simulink library "common_lib"  (R2023a)
settings: Solver=ode45  StartTime=0.0  StopTime=10.0  RelTol=1e-3
undefined symbols (not defined in the file): ACCEL_PRE_MULT, APDT_SrvcMgr_IRVHVDCSubFcnReq, C_C1GearNumbers, C_C1GearRatios, C_Calibration, C_DitherWaveform, C_GearOffset, C_GearRatioIn, C_GearRatioInverseOut, C_GearRatioOut, CLUTCH_INNER_LOOP_UPDATE_RATE, CONSTANT, DEGRADED_MODE_SIZE, Dem_EventStatusType, DiscIntNeverNeededParam, F_FAULT_ENUM, F_NOFAULT, F_OUTOFRANGE, F_RATELIMIT, FALSE, FMI14_SPECIAL_INSTRUCTIONS, FMI20_DATA_DRIFTED_HIGH, FMI21_DATA_DRIFTED_LOW, FMI29_RESERVED_FOR_SAE_ASSIGNMENT, FMI30_RESERVED_FOR_SAE_ASSIGNMENT, FMI31_CONDITION_EXISTS, FMI32_NO_FAULT, IC, k_accel, k_mean, MAX_UINT32, MEAN_PRE_MULT, NTriggers, QLTY_SIGNAL_FAILED, QLTY_SIGNAL_FULLY_FUNCTION, QLTY_SIGNAL_SUBSTITUTED_BY_1ST_CHOICE, QLTY_SIGNAL_SUBSTITUTED_BY_2ND_CHOICE, QLTY_SIGNAL_SUBSTITUTED_BY_3RD_CHOICE, QLTY_SIGNAL_SUBSTITUTED_BY_4TH_CHOICE, SAMPLE_TIME_100us, SAMPLETIME_10ms_Int, SATURATION_U16, simin, T_TestPoint, TF_FALSE, TF_TRUE, TimeStep, TRUE, WORKSPACE_UPDATE_RATE, ZERO, Zero
libraries: $bdroot x123, simulink x28, simulink_extras x4, MBD_EPS_Local_Blockset x4
(part 10 of 10)

== system common_lib/Signal Generators/Signal Generator Components/TestSignalPeriod ==
  TestSignalFrequency : Inport
  ClampAboveZero : $bdroot/Misc/ClampAboveZero  Tol=single(0.0001)
      settings: AttributesFormatString=tol=%<Tol>
  ClampAroundZero1 : $bdroot/Misc/ClampAroundZero  Tol=single(0.01)
      settings: AttributesFormatString=tol=%<Tol>
  Constant1 : Constant  Value=TimeStep  SampleTime=-1
  Constant35 : Constant  Value=single(2.0)  SampleTime=-1
  Constant39 : Constant  Value=single(1.0)  SampleTime=-1
  Data Type Conversion1 : DataTypeConversion  OutDataTypeStr=single  SaturateOnIntegerOverflow=off  RndMeth=Floor
  MinMax1 : MinMax  Function=max  Inputs=2  InputSameDT=on  ZeroCross=off
  Product15 : Product  Inputs=*/  OutDataTypeStr=Inherit: Same as first input
  Product19 : Product  Inputs=**  InputSameDT=on  OutDataTypeStr=Inherit: Same as first input
  TestSignalPeriod : Outport  VectorParamsAs1DForOutWhenUnconnected=off
  wires:
  Product15/1 -> MinMax1/1
  Constant39/1 -> Product15/1
  ClampAroundZero1/1 -> Product15/2
  TestSignalFrequency/1 -> ClampAroundZero1/1
  Constant1/1 -> Data Type Conversion1/1
  Constant35/1 -> Product19/2
  Product19/1 -> MinMax1/2
  MinMax1/1 -> TestSignalPeriod/1  "TestSignalPeriod"
  ClampAboveZero/1 -> Product19/1
  Data Type Conversion1/1 -> ClampAboveZero/1

== system common_lib/Signal Generators/Signal Generator Components/TestSignalPeriodTimer ==
  TestSignalReset : Inport
  TestSignalPeriod : Inport  Port=2
  ClampAboveZero : $bdroot/Misc/ClampAboveZero  Tol=single(0.0001)
      settings: AttributesFormatString=tol=%<Tol>
  Constant1 : Constant  Value=TimeStep  SampleTime=-1
  Constant40 : Constant  Value=false  SampleTime=-1
  Constant41 : Constant  Value=single(0.0)
  Data Type Conversion7 : DataTypeConversion  OutDataTypeStr=single  SaturateOnIntegerOverflow=off  RndMeth=Floor
  Logical Operator1 : Logic  Operator=OR  Inputs=3  AllPortsSameDT=off
  Relational Operator4 : RelationalOperator  ZeroCross=off  InputSameDT=off
  Sum5 : Sum  Inputs=2
  Switch5 : Switch  Threshold=0.5  ZeroCross=off  SaturateOnIntegerOverflow=off  InputSameDT=off
  Unit Delay4 : UnitDelay  InitialCondition=true  SampleTime=-1  HasFrameUpgradeWarning=on
      settings: AttributesFormatString=ic=%<X0>
  Unit Delay5 : UnitDelay  InitialCondition=single(0.0)  SampleTime=-1  HasFrameUpgradeWarning=on
      settings: AttributesFormatString=ic=%<X0>
  TestSignalTime : Outport  VectorParamsAs1DForOutWhenUnconnected=off
  wires:
  TestSignalReset/1 -> Logical Operator1/2
  Logical Operator1/1 -> Switch5/2
  Switch5/1 -> Unit Delay5/1, TestSignalTime/1  "TestSignalTime"
  Sum5/1 -> Switch5/3
  Constant41/1 -> Switch5/1
  Unit Delay4/1 -> Logical Operator1/1
  Constant40/1 -> Unit Delay4/1
  TestSignalPeriod/1 -> Relational Operator4/2
  Relational Operator4/1 -> Logical Operator1/3
  Unit Delay5/1 -> Relational Operator4/1, Sum5/1
  Constant1/1 -> Data Type Conversion7/1
  Data Type Conversion7/1 -> ClampAboveZero/1
  ClampAboveZero/1 -> Sum5/2

== system common_lib/Signal Generators/Signal Generator Components/TestSignalRamp ==
  TestSignalRampStart : Inport
  TestSignalRampEnd : Inport  Port=2
  TestSignalRampTime : Inport  Port=3
  TestSignalReset : Inport  Port=4
  Abs : Abs  ZeroCross=off  SaturateOnIntegerOverflow=off
  Constant35 : Constant  Value=single(0.01)  SampleTime=-1
  Logical Operator : Logic  AllPortsSameDT=off
  Logical Operator1 : Logic  Operator=NOT  AllPortsSameDT=off
  Logical Operator2 : Logic  Operator=NOT  AllPortsSameDT=off
  Logical Operator3 : Logic  Operator=OR  AllPortsSameDT=off
  Relational Operator : RelationalOperator  ZeroCross=off  InputSameDT=off
  Sum : Sum  Inputs=+-
  TestSignalRampEnabled : Subsystem
  Unit Delay : UnitDelay  InitialCondition=CLUTCH_INNER_LOOP_UPDATE_RATE  SampleTime=-1  HasFrameUpgradeWarning=on
      settings: AttributesFormatString=ic=%<X0>
  TestSignal : Outport  VectorParamsAs1DForOutWhenUnconnected=off
  wires:
  Logical Operator3/1 -> Logical Operator/2
  Logical Operator2/1 -> Logical Operator3/2
  Unit Delay/1 -> Logical Operator2/1
  Logical Operator1/1 -> Logical Operator3/1
  Logical Operator/1 -> TestSignalRampEnabled/Enable
  Relational Operator/1 -> Logical Operator/1
  Constant35/1 -> Relational Operator/2
  Abs/1 -> Relational Operator/1
  Sum/1 -> Abs/1
  TestSignalRampTime/1 -> TestSignalRampEnabled/3(TestSignalFreqRampTime)
  TestSignalRampEnabled/1(TestSignalFrequency) -> TestSignal/1
  TestSignalRampEnd/1 -> Sum/2, TestSignalRampEnabled/2(TestSignalFreqRampEnd)
  TestSignalRampStart/1 -> Sum/1, TestSignalRampEnabled/1(TestSignalFrequencyIn)
  TestSignalReset/1 -> Unit Delay/1, Logical Operator1/1, TestSignalRampEnabled/4(TestSignalReset)

== system common_lib/Signal Generators/Signal Generator Components/TestSignalSineWave ==
  TestSignalPk2PkAmplitude : Inport
  TestSignalOffset : Inport  Port=2
  TestSignalTime : Inport  Port=3
  TestSignalPeriod : Inport  Port=4
  TestSignalReset : Inport  Port=5
  Constant1 : Constant  Value=single(0.0)
  Data Type Conversion4 : DataTypeConversion  OutDataTypeStr=uint32  SaturateOnIntegerOverflow=off
  Look-Up Table : Lookup  InputValues=single([0 0.25 0.5 0.75 1])  Table=single([0 pi/2 0 -pi/2 0])  LookUpMeth=Interpolation-Use End Values  SaturateOnIntegerOverflow=off
      settings: AttributesFormatString=X=%<InputValues>\nY= %<OutputValues>
  Product1 : Product  Inputs=*/  OutDataTypeStr=Inherit: Same as first input
  Product16 : Product  Inputs=*/  OutDataTypeStr=Inherit: Same as first input
  Product18 : Product  Inputs=**  OutDataTypeStr=Inherit: Same as first input
  Sine1 : $bdroot/Misc/Sine
  Sum3 : Sum  Inputs=+-
  Sum4 : Sum
  Switch1 : Switch  Threshold=0.5  ZeroCross=off  SaturateOnIntegerOverflow=off  InputSameDT=off
  TestSignal : Outport  VectorParamsAs1DForOutWhenUnconnected=off
  wires:
  Sine1/1 -> Product18/1
  Look-Up Table/1 -> Sine1/1
  Product1/1 -> Look-Up Table/1  "TestSignalPeriodFrac"
  [TestSignalPeriod] -> Product1/2
  Switch1/1 -> Sum4/1
  Constant1/1 -> Switch1/1
  TestSignalReset/1 -> Switch1/2
  TestSignalPk2PkAmplitude/1 -> Product18/2
  TestSignalOffset/1 -> Sum4/2
  Sum4/1 -> TestSignal/1  "TestSignal"
  Product16/1 -> Sum3/1, Data Type Conversion4/1
  Data Type Conversion4/1 -> Sum3/2
  Sum3/1 -> Product1/1
  Product18/1 -> Switch1/3
  TestSignalTime/1 -> Product16/1, [TestSignalTime]
  TestSignalPeriod/1 -> Product16/2, [TestSignalPeriod]

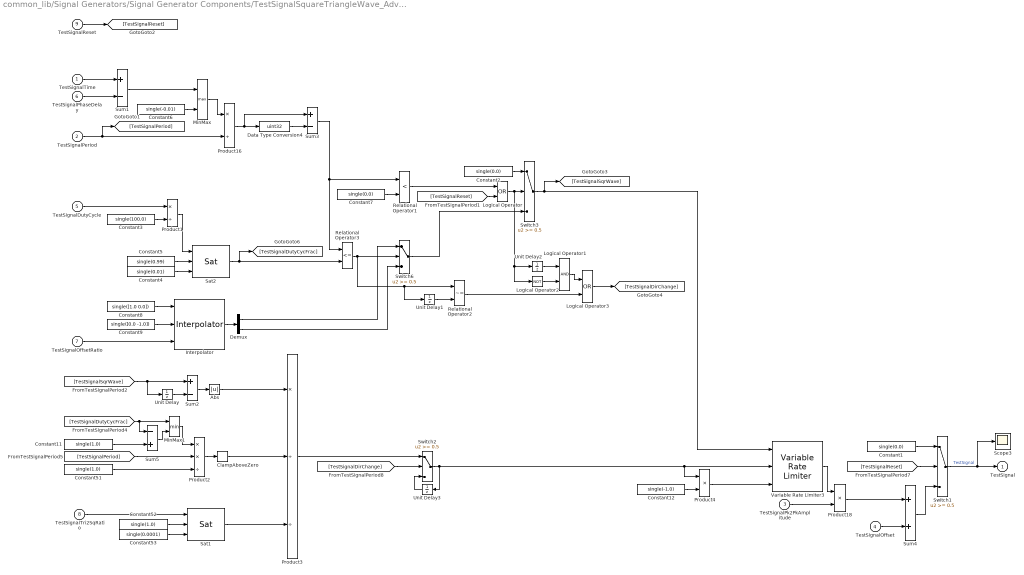
== system common_lib/Signal Generators/Signal Generator Components/TestSignalSquareTriangleWave_Advanced ==
  TestSignalTime : Inport
  TestSignalPeriod : Inport  Port=2
  TestSignalPk2PkAmplitude : Inport  Port=3
  TestSignalOffset : Inport  Port=4
  TestSignalDutyCycle : Inport  Port=5
  TestSignalPhaseDelay : Inport  Port=6
  TestSignalOffsetRatio : Inport  Port=7
  TestSignalTri2SqRatio : Inport  Port=8
  TestSignalReset : Inport  Port=9
  Abs : Abs  ZeroCross=off  SaturateOnIntegerOverflow=off
  ClampAboveZero : $bdroot/Misc/ClampAboveZero  Tol=single(0.001)
      settings: AttributesFormatString=tol=%<Tol>
  Constant1 : Constant  Value=single(0.0)
  Constant11 : Constant  Value=single(1.0)
  Constant12 : Constant  Value=single(-1.0)
  Constant2 : Constant  Value=single(0.0)
  Constant3 : Constant  Value=single(100.0)
  Constant4 : Constant  Value=single(0.01)
  Constant5 : Constant  Value=single(0.99)
  Constant51 : Constant  Value=single(1.0)
  Constant52 : Constant  Value=single(1.0)
  Constant53 : Constant  Value=single(0.0001)
  Constant6 : Constant  Value=single(-0.01)
  Constant7 : Constant  Value=single(0.0)
  Constant8 : Constant  Value=single([1.0 0.0])
  Constant9 : Constant  Value=single([0.0 -1.0])
  Data Type Conversion4 : DataTypeConversion  OutDataTypeStr=uint32  SaturateOnIntegerOverflow=off
  Demux : Demux  Outputs=2
  Interpolator : $bdroot/Tbl/Interpolator  DType=Single
  Logical Operator : Logic  Operator=OR  AllPortsSameDT=off
  Logical Operator1 : Logic  AllPortsSameDT=off
  Logical Operator2 : Logic  Operator=NOT  AllPortsSameDT=off
  Logical Operator3 : Logic  Operator=OR  AllPortsSameDT=off
  MinMax : MinMax  Function=max  Inputs=2  InputSameDT=on  ZeroCross=off
  MinMax1 : MinMax  Inputs=2  InputSameDT=on  ZeroCross=off
  Product1 : Product  Inputs=*/  OutDataTypeStr=Inherit: Same as first input
  Product16 : Product  Inputs=*/  OutDataTypeStr=Inherit: Same as first input
  Product18 : Product  Inputs=**  OutDataTypeStr=Inherit: Same as first input
  Product2 : Product  Inputs=**/  OutDataTypeStr=Inherit: Same as first input
  Product3 : Product  Inputs=*//  OutDataTypeStr=Inherit: Same as first input
  Product4 : Product  Inputs=**  OutDataTypeStr=Inherit: Same as first input
  Relational Operator1 : RelationalOperator  Operator=<  ZeroCross=off  InputSameDT=off
  Relational Operator2 : RelationalOperator  Operator=~=  ZeroCross=off  InputSameDT=off
  Relational Operator3 : RelationalOperator  Operator=<=  ZeroCross=off  InputSameDT=off
  Sat1 : $bdroot/Slink/Sat
  Sat2 : $bdroot/Slink/Sat
  Scope3 : Scope
  Sum1 : Sum  Inputs=+-
  Sum2 : Sum  Inputs=+-
  Sum3 : Sum  Inputs=+-
  Sum4 : Sum
  Sum5 : Sum  Inputs=-+
  Switch{1..3,6} (4 alike) : Switch  Threshold=0.5  ZeroCross=off  SaturateOnIntegerOverflow=off  InputSameDT=off
  Unit Delay : UnitDelay  InitialCondition=single(0.0)  SampleTime=-1  HasFrameUpgradeWarning=on
      settings: AttributesFormatString=ic=%<X0>
  Unit Delay1 : UnitDelay  InitialCondition=false  SampleTime=-1  HasFrameUpgradeWarning=on
      settings: AttributesFormatString=ic=%<X0>
  Unit Delay2 : UnitDelay  InitialCondition=false  SampleTime=-1  HasFrameUpgradeWarning=on
      settings: AttributesFormatString=ic=%<X0>
  Unit Delay3 : UnitDelay  InitialCondition=single(0.0)  SampleTime=-1  HasFrameUpgradeWarning=on
      settings: AttributesFormatString=ic=%<X0>
  Variable Rate Limiter3 : $bdroot/Slink/Variable Rate Limiter  TimeStep=TimeStep  ic=single(0.0)
  TestSignal : Outport  VectorParamsAs1DForOutWhenUnconnected=off
  wires:
  MinMax1/1 -> Product2/1
  Product4/1 -> Variable Rate Limiter3/3
  Constant12/1 -> Product4/2
  Abs/1 -> Product3/1
  [TestSignalDirChange] -> Switch2/2
  Unit Delay3/1 -> Switch2/3
  Switch2/1 -> Unit Delay3/1, Product4/1, Variable Rate Limiter3/2
  [TestSignalReset] -> Switch1/2
  Product3/1 -> Switch2/1
  Sum5/1 -> MinMax1/2
  Constant11/1 -> Sum5/2
  ClampAboveZero/1 -> Product3/2
  Sum2/1 -> Abs/1
  Product2/1 -> ClampAboveZero/1
  [TestSignalPeriod] -> Product2/2
  [TestSignalDutyCycFrac] -> MinMax1/1, Sum5/1
  Unit Delay/1 -> Sum2/2
  Logical Operator3/1 -> [TestSignalDirChange]
  Relational Operator2/1 -> Logical Operator3/2
  Logical Operator1/1 -> Logical Operator3/1
  Logical Operator2/1 -> Logical Operator1/2
  Unit Delay2/1 -> Logical Operator1/1
  Unit Delay1/1 -> Relational Operator2/2
  [TestSignalSqrWave] -> Sum2/1, Unit Delay/1
  Logical Operator/1 -> Logical Operator2/1, Unit Delay2/1, Switch3/2
  [TestSignalReset] -> Logical Operator/2
  Demux/2 -> Switch6/3
  Demux/1 -> Switch6/1
  Interpolator/1 -> Demux/1
  Constant2/1 -> Switch3/1
  Constant8/1 -> Interpolator/1
  Switch3/1 -> [TestSignalSqrWave], Variable Rate Limiter3/1
  Constant9/1 -> Interpolator/2
  TestSignalOffsetRatio/1 -> Interpolator/3
  Relational Operator1/1 -> Logical Operator/1
  Constant7/1 -> Relational Operator1/2
  MinMax/1 -> Product16/1
  Constant6/1 -> MinMax/2
  TestSignalPhaseDelay/1 -> Sum1/2
  Sum1/1 -> MinMax/1
  Sat2/1 -> [TestSignalDutyCycFrac], Relational Operator3/2
  Constant5/1 -> Sat2/2
  Constant4/1 -> Sat2/3
  Product1/1 -> Sat2/1
  Constant3/1 -> Product1/2
  TestSignalDutyCycle/1 -> Product1/1
  Switch1/1 -> Scope3/1, TestSignal/1  "TestSignal"
  Constant1/1 -> Switch1/1
  Sat1/1 -> Product3/3
  Constant53/1 -> Sat1/3
  Constant52/1 -> Sat1/2
  TestSignalTri2SqRatio/1 -> Sat1/1
  Constant51/1 -> Product2/3
  Variable Rate Limiter3/1 -> Product18/1
  TestSignalPk2PkAmplitude/1 -> Product18/2
  TestSignalOffset/1 -> Sum4/2
  Product16/1 -> Sum3/1, Data Type Conversion4/1
  Data Type Conversion4/1 -> Sum3/2
  Sum3/1 -> Relational Operator1/1, Relational Operator3/1
  Relational Operator3/1 -> Unit Delay1/1, Relational Operator2/1, Switch6/2
  Switch6/1 -> Switch3/3
  Product18/1 -> Sum4/1
  TestSignalTime/1 -> Sum1/1
  TestSignalPeriod/1 -> Product16/2, [TestSignalPeriod]
  Sum4/1 -> Switch1/3
  TestSignalReset/1 -> [TestSignalReset]

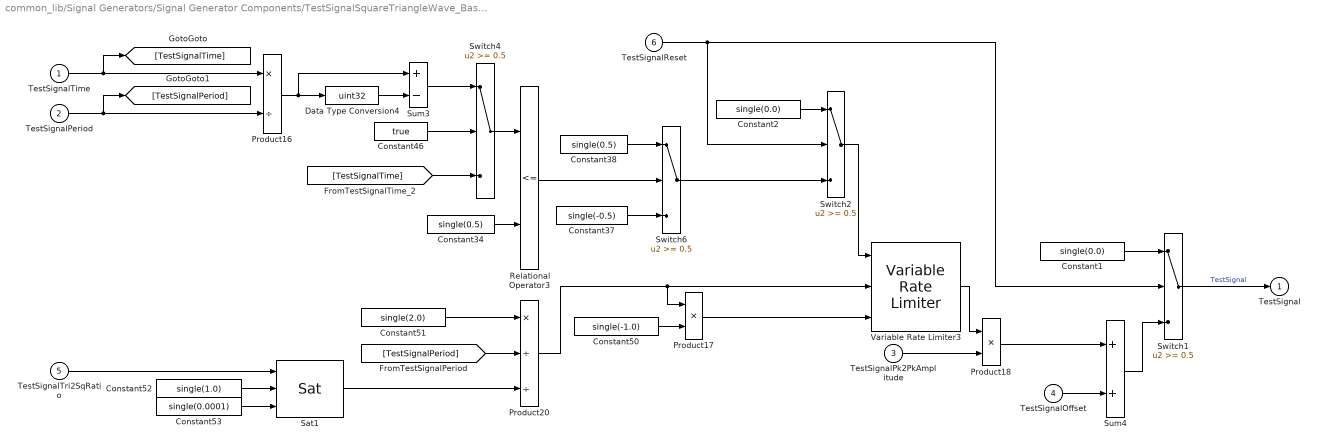
== system common_lib/Signal Generators/Signal Generator Components/TestSignalSquareTriangleWave_Basic ==
  TestSignalTime : Inport
  TestSignalPeriod : Inport  Port=2
  TestSignalPk2PkAmplitude : Inport  Port=3
  TestSignalOffset : Inport  Port=4
  TestSignalTri2SqRatio : Inport  Port=5
  TestSignalReset : Inport  Port=6
  Constant1 : Constant  Value=single(0.0)
  Constant2 : Constant  Value=single(0.0)
  Constant34 : Constant  Value=single(0.5)  SampleTime=-1
  Constant37 : Constant  Value=single(-0.5)  SampleTime=-1
  Constant38 : Constant  Value=single(0.5)  SampleTime=-1
  Constant46 : Constant  Value=true  SampleTime=-1
  Constant50 : Constant  Value=single(-1.0)
  Constant51 : Constant  Value=single(2.0)
  Constant52 : Constant  Value=single(1.0)
  Constant53 : Constant  Value=single(0.0001)
  Data Type Conversion4 : DataTypeConversion  OutDataTypeStr=uint32  SaturateOnIntegerOverflow=off
  Product16 : Product  Inputs=*/  OutDataTypeStr=Inherit: Same as first input
  Product17 : Product  Inputs=**  OutDataTypeStr=Inherit: Same as first input
  Product18 : Product  Inputs=**  OutDataTypeStr=Inherit: Same as first input
  Product20 : Product  Inputs=*//  OutDataTypeStr=Inherit: Same as first input
  Relational Operator3 : RelationalOperator  Operator=<=  ZeroCross=off  InputSameDT=off
  Sat1 : $bdroot/Slink/Sat
  Sum3 : Sum  Inputs=+-
  Sum4 : Sum
  Switch{1..2,4,6} (4 alike) : Switch  Threshold=0.5  ZeroCross=off  SaturateOnIntegerOverflow=off  InputSameDT=off
  Variable Rate Limiter3 : $bdroot/Slink/Variable Rate Limiter  TimeStep=TimeStep  ic=single(0.0)
  TestSignal : Outport  VectorParamsAs1DForOutWhenUnconnected=off
  wires:
  Switch2/1 -> Variable Rate Limiter3/1
  Constant2/1 -> Switch2/1
  TestSignalReset/1 -> Switch1/2, Switch2/2
  Sum4/1 -> Switch1/3
  TestSignalPeriod/1 -> [TestSignalPeriod], Product16/2
  TestSignalTime/1 -> [TestSignalTime], Product16/1
  Product18/1 -> Sum4/1
  Switch6/1 -> Switch2/3
  Constant38/1 -> Switch6/1
  Constant37/1 -> Switch6/3
  Relational Operator3/1 -> Switch6/2
  Switch4/1 -> Relational Operator3/1
  [TestSignalTime] -> Switch4/3
  Constant46/1 -> Switch4/2
  Sum3/1 -> Switch4/1
  Data Type Conversion4/1 -> Sum3/2
  Product16/1 -> Data Type Conversion4/1, Sum3/1
  Constant34/1 -> Relational Operator3/2
  TestSignalOffset/1 -> Sum4/2
  TestSignalPk2PkAmplitude/1 -> Product18/2
  Product20/1 -> Product17/1, Variable Rate Limiter3/2
  Product17/1 -> Variable Rate Limiter3/3
  Constant50/1 -> Product17/2
  Variable Rate Limiter3/1 -> Product18/1
  Constant51/1 -> Product20/1
  [TestSignalPeriod] -> Product20/2
  TestSignalTri2SqRatio/1 -> Sat1/1
  Constant52/1 -> Sat1/2
  Constant53/1 -> Sat1/3
  Sat1/1 -> Product20/3
  Constant1/1 -> Switch1/1
  Switch1/1 -> TestSignal/1  "TestSignal"

== system common_lib/Signal Generators/Signal Generator Components/TestSignalTimer ==
  TestSignalReset : Inport
  Constant1 : Constant  Value=TimeStep  SampleTime=-1
  Constant40 : Constant  Value=false  SampleTime=-1
  Constant41 : Constant  Value=single(0.0)
  Constant43 : Constant  Value=single(1000000)
  Data Type Conversion7 : DataTypeConversion  OutDataTypeStr=single  SaturateOnIntegerOverflow=off  RndMeth=Floor
  Logical Operator1 : Logic  Operator=OR  Inputs=3  AllPortsSameDT=off
  Relational Operator4 : RelationalOperator  ZeroCross=off  InputSameDT=off
  Sum5 : Sum  Inputs=2
  Switch5 : Switch  Threshold=0.5  ZeroCross=off  SaturateOnIntegerOverflow=off  InputSameDT=off
  Unit Delay4 : UnitDelay  InitialCondition=true  SampleTime=-1  HasFrameUpgradeWarning=on
      settings: AttributesFormatString=ic=%<X0>
  Unit Delay5 : UnitDelay  InitialCondition=single(0.0)  SampleTime=-1  HasFrameUpgradeWarning=on
      settings: AttributesFormatString=ic=%<X0>
  TestSignalTime : Outport  VectorParamsAs1DForOutWhenUnconnected=off
  wires:
  Constant1/1 -> Data Type Conversion7/1
  TestSignalReset/1 -> Logical Operator1/2
  Logical Operator1/1 -> Switch5/2
  Switch5/1 -> Unit Delay5/1, TestSignalTime/1  "TestSignalTime"
  Sum5/1 -> Switch5/3
  Constant41/1 -> Switch5/1
  Unit Delay4/1 -> Logical Operator1/1
  Constant40/1 -> Unit Delay4/1
  Constant43/1 -> Relational Operator4/2
  Relational Operator4/1 -> Logical Operator1/3
  Unit Delay5/1 -> Relational Operator4/1, Sum5/1
  Data Type Conversion7/1 -> Sum5/2

== system common_lib/Tbl/XY Interpolator1/XYInterp ==
  y_value_1 : Inport
  y_value_0 : Inport  Port=2
  x_value_1 : Inport  Port=3
  x_value_0 : Inport  Port=4
  x_value : Inport  Port=5
  ClampAroundZero : $bdroot/Misc/ClampAroundZero  Tol=Tol
  Constant1 : Constant  Value=Zero
  Constant2 : Constant  Value=One
  Product1 : Product  Inputs=*/  InputSameDT=on  OutDataTypeStr=Inherit: Same as first input
  Product2 : Product  Inputs=**  InputSameDT=on  OutDataTypeStr=Inherit: Same as first input
  Sat : $bdroot/Slink/Sat
  Sum : Sum  Inputs=+-  InputSameDT=on  OutDataTypeStr=Inherit: Same as first input
  Sum1 : Sum  Inputs=|++  InputSameDT=on  OutDataTypeStr=Inherit: Same as first input
  Sum2 : Sum  Inputs=-+  InputSameDT=on  OutDataTypeStr=Inherit: Same as first input
  Sum3 : Sum  Inputs=+-  InputSameDT=on  OutDataTypeStr=Inherit: Same as first input
  output : Outport  VectorParamsAs1DForOutWhenUnconnected=off
  wires:
  y_value_0/1 -> Sum1/2, Sum/2
  y_value_1/1 -> Sum/1
  Sum1/1 -> output/1
  Product2/1 -> Sum1/1
  Sum/1 -> Product2/1
  x_value/1 -> Sum3/1
  x_value_0/1 -> Sum3/2, Sum2/1
  Sum3/1 -> Product1/1
  x_value_1/1 -> Sum2/2
  Sum2/1 -> ClampAroundZero/1
  ClampAroundZero/1 -> Product1/2
  Product1/1 -> Sat/1
  Sat/1 -> Product2/2
  Constant2/1 -> Sat/2
  Constant1/1 -> Sat/3

== system common_lib/Diagnostics/Calibration Enabled MinMax OOR/Enabled OOR/OOR MinMax Capture ==
  Input : Inport
  Hold : Inport  Port=2
  Enable : EnablePort  ZeroCross=off
  CL MinMax Capture : $bdroot/Diag/CL MinMax Capture  CaptureType=Max  InDataType=single
  CL MinMax Capture1 : $bdroot/Diag/CL MinMax Capture  CaptureType=Min  InDataType=single
  DRDataStoreRead : DataStoreRead  DataStoreName=InitializeStates  IndexOptions=Index vector (dialog)  Indices=1  OutputSizes=1
  Max : Outport  VectorParamsAs1DForOutWhenUnconnected=off
  Min : Outport  Port=2  VectorParamsAs1DForOutWhenUnconnected=off
  wires:
  Input/1 -> CL MinMax Capture1/1, CL MinMax Capture/1
  Hold/1 -> CL MinMax Capture1/2, CL MinMax Capture/2
  DRDataStoreRead/1 -> CL MinMax Capture/3, CL MinMax Capture1/3
  CL MinMax Capture/1 -> Max/1
  CL MinMax Capture1/1 -> Min/1

== system common_lib/Diagnostics/Calibration Enabled MinMax RLim/Enabled RLim/RLim MinMax Capture ==
  Input : Inport
  Hold : Inport  Port=2
  Enable : EnablePort  ZeroCross=off
  CL MinMax Capture : $bdroot/Diag/CL MinMax Capture  CaptureType=Max  InDataType=single
  CL MinMax Capture1 : $bdroot/Diag/CL MinMax Capture  CaptureType=Min  InDataType=single
  DRDataStoreRead : DataStoreRead  DataStoreName=InitializeStates  IndexOptions=Index vector (dialog)  Indices=1  OutputSizes=1
  Sum1 : Sum  Inputs=|+-  InputSameDT=on  OutDataTypeStr=Inherit: Same as first input
  Unit Delay2 : UnitDelay  InitialCondition=Zero  SampleTime=-1  HasFrameUpgradeWarning=on
      settings: AttributesFormatString=ic=%<X0>
  Max : Outport  VectorParamsAs1DForOutWhenUnconnected=off
  Min : Outport  Port=2  VectorParamsAs1DForOutWhenUnconnected=off
  wires:
  Input/1 -> Sum1/1, Unit Delay2/1
  Hold/1 -> CL MinMax Capture1/2, CL MinMax Capture/2
  CL MinMax Capture/1 -> Max/1
  CL MinMax Capture1/1 -> Min/1
  Unit Delay2/1 -> Sum1/2
  Sum1/1 -> CL MinMax Capture1/1, CL MinMax Capture/1
  DRDataStoreRead/1 -> CL MinMax Capture/3, CL MinMax Capture1/3

== system common_lib/Diagnostics/Calibration Enabled MinMax RLim/Enabled RLim/RateLimit ==
  in : Inport
  rlim : Inport  Port=2
  ext_fault? : Inport  Port=3
  Constant2 : Constant  Value=TimeStep
  DRDataStoreRead : DataStoreRead  DataStoreName=InitializeStates  IndexOptions=Index vector (dialog)  Indices=1  OutputSizes=1
  Data Type Conversion : DataTypeConversion  OutDataTypeStr=single  SaturateOnIntegerOverflow=off  RndMeth=Floor
  Logical Operator : Logic  Operator=NOT
  OOR Fault Detection : $bdroot/Diag/OOR Fault Detection  InitialValue=IC
  Product1 : Product  InputSameDT=on  OutDataTypeStr=Inherit: Same as first input
  Sum1 : Sum  Inputs=-+|  InputSameDT=on  OutDataTypeStr=Inherit: Same as first input
  Sum2 : Sum  Inputs=|++  InputSameDT=on  OutDataTypeStr=Inherit: Same as first input
  Sum3 : Sum  Inputs=++|  InputSameDT=on  OutDataTypeStr=Inherit: Same as first input
  Unit Delay : UnitDelay  InitialCondition=Zero  SampleTime=-1  HasFrameUpgradeWarning=on
      settings: AttributesFormatString=ic=%<X0>
  Unit Delay1 : UnitDelay  InitialCondition=false  SampleTime=-1  HasFrameUpgradeWarning=on
      settings: AttributesFormatString=ic=%<X0>
  Unit Delay2 : UnitDelay  InitialCondition=Zero  SampleTime=-1  HasFrameUpgradeWarning=on
      settings: AttributesFormatString=ic=%<X0>
  inc switch : Switch  Threshold=0.5  ZeroCross=off  SaturateOnIntegerOverflow=off
  inc switch1 : Switch  Threshold=0.5  ZeroCross=off  SaturateOnIntegerOverflow=off
  out : Outport  VectorParamsAs1DForOutWhenUnconnected=off
  fault? : Outport  Port=2  VectorParamsAs1DForOutWhenUnconnected=off
  wires:
  Constant2/1 -> Data Type Conversion/1
  Data Type Conversion/1 -> Product1/1
  inc switch1/1 -> Sum2/1, Sum1/2
  Unit Delay/1 -> inc switch1/1
  Unit Delay1/1 -> inc switch/2
  Unit Delay2/1 -> Sum3/1
  Sum3/1 -> inc switch/1
  Product1/1 -> Sum3/2, inc switch/3
  rlim/1 -> Product1/2
  inc switch/1 -> Unit Delay2/1, Sum1/1, Sum2/2
  Sum2/1 -> OOR Fault Detection/2
  Sum1/1 -> OOR Fault Detection/3
  OOR Fault Detection/2 -> Unit Delay1/1, fault?/1
  OOR Fault Detection/1 -> Unit Delay/1, out/1
  ext_fault?/1 -> OOR Fault Detection/4
  in/1 -> inc switch1/3, OOR Fault Detection/1
  DRDataStoreRead/1 -> Logical Operator/1
  Logical Operator/1 -> inc switch1/2

== system common_lib/OS/Scheduler with Init/Init Relay/Function Call ==
  InitActive : EnablePort  StatesWhenEnabling=reset  ZeroCross=off
  Function-Call Generator : simulink/Ports & Subsystems/Function-Call Generator  sample_time=-1  numberOfIterations=1  DisallowWideOutput=off
  Init : Outport  VectorParamsAs1DForOutWhenUnconnected=off
  wires:
  Function-Call Generator/1 -> Init/1

== system common_lib/Signal Generators/Signal Generator Components/TestSignalRamp/TestSignalRampEnabled ==
  TestSignalFrequencyIn : Inport
  TestSignalFreqRampEnd : Inport  Port=2
  TestSignalFreqRampTime : Inport  Port=3
  TestSignalReset : Inport  Port=4
  Enable : EnablePort  StatesWhenEnabling=reset  ZeroCross=off
  Ramp : $bdroot/Ctrl/Ramp  TimeStep=TimeStep
  TestSignalFrequency : Outport  VectorParamsAs1DForOutWhenUnconnected=off
  wires:
  Ramp/1 -> TestSignalFrequency/1
  TestSignalReset/1 -> Ramp/4
  TestSignalFreqRampTime/1 -> Ramp/3
  TestSignalFreqRampEnd/1 -> Ramp/2
  TestSignalFrequencyIn/1 -> Ramp/1

== stateflow chart common_lib/Bit/uint8 Bit Pack ==
  settings: stateMachineType=MEALY_MACHINE
  (default) -> (junction 10) : {Byte=0;}
  (junction 10) -> (junction 13) [order 1] : [Bit_0]{Byte=Byte | 1;}
  (junction 10) -> (junction 13) [order 2]
  (junction 13) -> (junction 20) [order 1] : [Bit_1]{Byte=Byte | 2;}
  (junction 13) -> (junction 20) [order 2]
  (junction 20) -> (junction 26) [order 1] : [Bit_2]{Byte=Byte | 4;}
  (junction 20) -> (junction 26) [order 2]
  (junction 26) -> (junction 31) [order 1] : [Bit_3]{Byte=Byte | 8;}
  (junction 26) -> (junction 31) [order 2]
  (junction 31) -> (junction 36) [order 1] : [Bit_4]{Byte=Byte | 16;}
  (junction 31) -> (junction 36) [order 2]
  (junction 36) -> (junction 41) [order 1] : [Bit_5]{Byte=Byte | 32;}
  (junction 36) -> (junction 41) [order 2]
  (junction 41) -> (junction 46) [order 1] : [Bit_6]{Byte=Byte | 64;}
  (junction 41) -> (junction 46) [order 2]
  (junction 46) -> (junction 51) [order 1] : [Bit_7]{Byte=Byte | 128;}
  (junction 46) -> (junction 51) [order 2]
  data: Bit_0 input boolean size=1; Bit_1 input boolean size=1; Bit_2 input boolean size=1; Bit_3 input boolean size=1; Bit_4 input boolean size=1; Bit_5 input boolean size=1; Bit_6 input boolean size=1; Bit_7 input boolean size=1; Byte output uint8 size=1

== stateflow chart common_lib/Bit/uint8 Bit Unpack ==
  settings: stateMachineType=MEALY_MACHINE
  (default) -> (junction 17) : {Bit_0 = Byte & 1;
      |  Bit_1 = Byte & 2;
      |  Bit_2 = Byte & 4;
      |  Bit_3 = Byte & 8;
      |  Bit_4 = Byte & 16;
      |  Bit_5 = Byte & 32;
      |  Bit_6 = Byte & 64;
      |  Bit_7 = Byte & 128;}
  data: Byte input uint8 size=1; Bit_0 output boolean size=1; Bit_1 output boolean size=1; Bit_2 output boolean size=1; Bit_3 output boolean size=1; Bit_4 output boolean size=1; Bit_5 output boolean size=1; Bit_6 output boolean size=1; Bit_7 output boolean size=1

== stateflow chart common_lib/Bit/uint16 Bit Pack ==
  settings: stateMachineType=MEALY_MACHINE
  (default) -> (junction 10) : {Byte=0;}
  (junction 10) -> (junction 13) [order 1] : [Bit_0]{Byte=Byte | 1;}
  (junction 10) -> (junction 13) [order 2]
  (junction 13) -> (junction 20) [order 1] : [Bit_1]{Byte=Byte | 2;}
  (junction 13) -> (junction 20) [order 2]
  (junction 20) -> (junction 26) [order 1] : [Bit_2]{Byte=Byte | 4;}
  (junction 20) -> (junction 26) [order 2]
  (junction 26) -> (junction 31) [order 1] : [Bit_3]{Byte=Byte | 8;}
  (junction 26) -> (junction 31) [order 2]
  (junction 31) -> (junction 36) [order 1] : [Bit_4]{Byte=Byte | 16;}
  (junction 31) -> (junction 36) [order 2]
  (junction 36) -> (junction 41) [order 1] : [Bit_5]{Byte=Byte | 32;}
  (junction 36) -> (junction 41) [order 2]
  (junction 41) -> (junction 46) [order 1] : [Bit_6]{Byte=Byte | 64;}
  (junction 41) -> (junction 46) [order 2]
  (junction 46) -> (junction 65) [order 1] : [Bit_7]{Byte=Byte | 128;}
  (junction 46) -> (junction 65) [order 2]
  (junction 65) -> (junction 66) [order 1] : [Bit_8]{Byte=Byte | 256;}
  (junction 65) -> (junction 66) [order 2]
  (junction 66) -> (junction 69) [order 1] : [Bit_9]{Byte=Byte | 512;}
  (junction 66) -> (junction 69) [order 2]
  (junction 69) -> (junction 72) [order 1] : [Bit_10]{Byte=Byte | 1024;}
  (junction 69) -> (junction 72) [order 2]
  (junction 72) -> (junction 73) [order 1] : [Bit_11]{Byte=Byte | 2048;}
  (junction 72) -> (junction 73) [order 2]
  (junction 73) -> (junction 68) [order 1] : [Bit_12]{Byte=Byte | 4096;}
  (junction 73) -> (junction 68) [order 2]
  (junction 68) -> (junction 71) [order 1] : [Bit_13]{Byte=Byte | 8192;}
  (junction 68) -> (junction 71) [order 2]
  (junction 71) -> (junction 70) [order 1] : [Bit_14]{Byte=Byte | 16384;}
  (junction 71) -> (junction 70) [order 2]
  (junction 70) -> (junction 67) [order 1] : [Bit_15]{Byte=Byte | 32768;}
  (junction 70) -> (junction 67) [order 2]
  data: Bit_0 input boolean size=1; Bit_1 input boolean size=1; Bit_2 input boolean size=1; Bit_3 input boolean size=1; Bit_4 input boolean size=1; Bit_5 input boolean size=1; Bit_6 input boolean size=1; Bit_7 input boolean size=1; Byte output uint16 size=1; Bit_8 input boolean size=1; Bit_9 input boolean size=1; Bit_10 input boolean size=1; Bit_11 input boolean size=1; Bit_12 input boolean size=1; Bit_13 input boolean size=1; Bit_14 input boolean size=1; Bit_15 input boolean size=1

== stateflow chart common_lib/Bit/uint16 Bit Unpack ==
  settings: stateMachineType=MEALY_MACHINE
  (default) -> (junction 17) : {Bit_0 = Byte & 1;
      |  Bit_1 = Byte & 2;
      |  Bit_2 = Byte & 4;
      |  Bit_3 = Byte & 8;
      |  Bit_4 = Byte & 16;
      |  Bit_5 = Byte & 32;
      |  Bit_6 = Byte & 64;
      |  Bit_7 = Byte & 128;
      |  Bit_8 = Byte & 256;
      |  Bit_9 = Byte & 512;
      |  Bit_10 = Byte & 1024;
      |  Bit_11 = Byte & 2048;
      |  Bit_12 = Byte & 4096;
      |  Bit_13 = Byte & 8192;
      |  Bit_14 = Byte & 16384;
      |  Bit_15 = Byte & 32768;}
  data: Byte input uint16 size=1; Bit_0 output boolean size=1; Bit_1 output boolean size=1; Bit_2 output boolean size=1; Bit_3 output boolean size=1; Bit_4 output boolean size=1; Bit_5 output boolean size=1; Bit_6 output boolean size=1; Bit_7 output boolean size=1; Bit_8 output boolean size=1; Bit_9 output boolean size=1; Bit_10 output boolean size=1; Bit_11 output boolean size=1; Bit_12 output boolean size=1; Bit_13 output boolean size=1; Bit_14 output boolean size=1; Bit_15 output boolean size=1

== stateflow chart common_lib/Diagnostics/DiagFaultCounter/DiagFaulCounter ==
  state FaultDebounceDisabled
    en: diagFaultStatus = Dem_EventStatusType.DEM_EVENT_STATUS_INIT;
    diagFaultCnt = int16(0);
    FaultDebounceDisabled -> (junction 32) [order 1]
    (junction 32) -> (junction 29) [order 1] : [~diagStartUpComp || diagReset || ~diagEnable]
        | {diagFaultStatus = Dem_EventStatusType.DEM_EVENT_STATUS_INIT;}
    (junction 32) -> (junction 23) [order 2]
    (junction 29) -> (junction 27)
    (junction 23) -> (junction 24) [order 1] : [~diagFaultActive]
        | {diagFaultStatus = Dem_EventStatusType.DEM_EVENT_STATUS_PREPASSED;}
    (junction 23) -> (junction 26) [order 2]
    (junction 24) -> (junction 282)
    (junction 26) -> (junction 281) [order 1] : [diagFaultActive]
        | {diagFaultStatus = Dem_EventStatusType.DEM_EVENT_STATUS_PREFAILED;}
    (junction 26) -> (junction 51) [order 2]
    (junction 281) -> (junction 283)
    (junction 283) -> (junction 51)
    (junction 282) -> (junction 283)
    (junction 27) -> (junction 282)
    (junction 51) -> (junction 288)
  state FaultDebounceEnabled
    en: diagFaultStatus = Dem_EventStatusType.DEM_EVENT_STATUS_INIT;
    diagFaultCnt = int16(0);
    state Init
      en: diagFaultCnt = int16(0);
      diagFaultStatus = Dem_EventStatusType.DEM_EVENT_STATUS_INIT;
      Init -> (junction 248) [order 1]
      (junction 248) -> (junction 249) [order 1] : [~diagStartUpComp || diagReset || ~diagEnable]
          | {diagFaultCnt = int16(0);}
      (junction 248) -> (junction 250) [order 2]
      (junction 249) -> (junction 257)
      (junction 250) -> (junction 253) [order 1] : [~diagFaultActive]
          | {diagFaultCnt = diagFaultCnt - diagDnCnt;}
      (junction 253) -> (junction 342) [order 1] : [diagFaultCnt<=diagPassCntThresh]
          | {diagFaultStatus = Dem_EventStatusType.DEM_EVENT_STATUS_PASSED;}
      (junction 250) -> (junction 252) [order 2]
      (junction 253) -> (junction 255) [order 2]
      (junction 342) -> (junction 344)
      (junction 252) -> (junction 251) [order 1] : [diagFaultActive]
          | {diagFaultCnt = diagFaultCnt + diagUpCnt;}
      (junction 251) -> (junction 310) [order 1] : [diagFaultCnt>=diagFaultCntThresh]
          | {diagFaultStatus = Dem_EventStatusType.DEM_EVENT_STATUS_FAILED;}
      (junction 251) -> (junction 256) [order 2]
      (junction 310) -> (junction 338)
      (junction 252) -> (junction 254) [order 2]
      (junction 256) -> (junction 254)
      (junction 338) -> (junction 256)
      (junction 255) -> (junction 338)
      (junction 344) -> (junction 255)
      (junction 257) -> (junction 344)
      (junction 254) -> (junction 258)
    state Fault
      en: diagFaultCnt = int16(0);
      diagFaultStatus = Dem_EventStatusType.DEM_EVENT_STATUS_FAILED;
      Fault -> (junction 133) [order 1]
      (junction 133) -> (junction 134) [order 1] : [(diagFaultCnt<int16(0)) && diagFaultActive]
          | {diagFaultCnt = diagFaultCnt + diagUpCnt;}
      (junction 134) -> (junction 152) [order 1] : [diagFaultCnt>int16(0)]
          | {diagFaultCnt = int16(0)}
      (junction 133) -> (junction 135) [order 2]
      (junction 134) -> (junction 139) [order 2]
      (junction 152) -> (junction 155)
      (junction 135) -> (junction 136) [order 1] : [~diagFaultActive && diagHealEn]
          | {diagFaultCnt = diagFaultCnt - diagDnCnt;}
      (junction 136) -> (junction 298) [order 1] : [diagFaultCnt<=diagPassCntThresh]
          | {diagFaultStatus = Dem_EventStatusType.DEM_EVENT_STATUS_PASSED;}
      (junction 135) -> (junction 137) [order 2]
      (junction 136) -> (junction 138) [order 2]
      (junction 298) -> (junction 300)
      (junction 138) -> (junction 137)
      (junction 300) -> (junction 138)
      (junction 139) -> (junction 300)
      (junction 155) -> (junction 139)
      (junction 137) -> (junction 140)
    state Pass
      en: diagFaultCnt = int16(0);
      diagFaultStatus = Dem_EventStatusType.DEM_EVENT_STATUS_PASSED;
      Pass -> (junction 159) [order 1]
      (junction 159) -> (junction 160) [order 1] : [(diagFaultCnt>int16(0)) && ~diagFaultActive]
          | {diagFaultCnt = diagFaultCnt - diagDnCnt;}
      (junction 160) -> (junction 161) [order 1] : [diagFaultCnt<int16(0)]
          | {diagFaultCnt = int16(0)}
      (junction 159) -> (junction 162) [order 2]
      (junction 160) -> (junction 166) [order 2]
      (junction 161) -> (junction 167)
      (junction 162) -> (junction 163) [order 1] : [diagFaultActive]
          | {diagFaultCnt = diagFaultCnt + diagUpCnt;}
      (junction 163) -> (junction 305) [order 1] : [diagFaultCnt>=diagFaultCntThresh]
          | {diagFaultStatus = Dem_EventStatusType.DEM_EVENT_STATUS_FAILED;}
      (junction 162) -> (junction 164) [order 2]
      (junction 163) -> (junction 165) [order 2]
      (junction 305) -> (junction 304)
      (junction 165) -> (junction 164)
      (junction 304) -> (junction 165)
      (junction 166) -> (junction 304)
      (junction 167) -> (junction 166)
      (junction 164) -> (junction 168)
    (default) -> Init
    Init -> Fault [order 1] : [diagFaultCnt>=diagFaultCntThresh &&...
        | diagStartUpComp &&...
        | ~diagReset && diagEnable]
    Fault -> Init [order 2] : [~diagStartUpComp ||...
        | diagReset || ~diagEnable]
    Fault -> Pass [order 1] : [diagFaultCnt<=diagPassCntThresh && diagHealEn]
    Pass -> Fault [order 1] : [diagFaultCnt>=diagFaultCntThresh]
    Init -> Pass [order 2] : [diagFaultCnt<=diagPassCntThresh &&...
        | diagStartUpComp &&...
        | ~diagReset && diagEnable]
    Pass -> Init [order 2] : [~diagStartUpComp ||...
        | diagReset || ~diagEnable]
  (default) -> (junction 58)
  (junction 58) -> (junction 279) [order 2]
  (junction 58) -> FaultDebounceEnabled [order 1] : [diagDbncEnab]
  (junction 279) -> FaultDebounceDisabled
  FaultDebounceEnabled -> FaultDebounceDisabled : [~diagDbncEnab]
  FaultDebounceDisabled -> FaultDebounceEnabled [order 1] : [diagDbncEnab]
  data: diagFaultActive input boolean size=1; diagStartUpComp input boolean size=1; diagReset input boolean size=1; diagEnable input boolean size=1; diagDbncEnab input boolean size=1; diagFaultCntThresh input int16 size=1; diagPassCntThresh input int16 size=1; diagUpCnt input int16 size=1; diagDnCnt input int16 size=1; diagFaultStatus output size=1; diagHealEn input boolean size=1; diagFaultCnt local int16 size=1
